simulink model "real_time_6"  (R2024b)
settings: Solver=FixedStepDiscrete  StartTime=0.0  StopTime=5  FixedStep=0.001  RelTol=1e-3
values from neighbouring files (symbols this model uses):
  AF = REG_disc.A    [code_ali.m]
  BF = REG_disc.B    [code_ali.m]
  CF = REG_disc.C    [code_ali.m]
  DF = REG_disc.D    [code_ali.m]
  K2 = K_robust(2:3)    [Pos_state_space.m]    (also in code_ali.m)
  KI = K_robust(1)    [Pos_state_space.m]    (also in code_ali.m)
  Nu = Ans(3,1)    [Pos_state_space.m]    (also in code_ali.m)
  Nx = Ans(1:2,1)    [Pos_state_space.m]    (also in code_ali.m)
  T_s = 0.001*10    (= 0.01)    [code_ali.m]
undefined symbols (not defined in the file or in its folder): degs2rpm, DiscIntNeverNeededParam, National_Instruments, PCI, rpm2rads
libraries: sldrtlib x3
settings Model: SimulationMode=external  ExtModeTrigDuration=1000001  Creator=galeazzolu  LastModifiedBy=galeazzolu
settings DataIOCC: ReturnWorkspaceOutputs=off
settings HardwareCC: ProdBitPerLong=64  ProdHWDeviceType=Intel->x86-64 (Linux 64)
settings RTWCC: Description=Simulink Desktop Real-Time  SystemTargetFile=sldrt.tlc  TemplateMakefile=sldrt.tmf  RTWCompilerOptimization=on
settings CodeAppCC: MaxIdLength=95
settings SimulinkDesktopRealTimeCC: TargetLibSuffix=_sldrt.a  TargetPreCompLibLocation=C:\Program Files\MATLAB\R2024b\toolbox\sldrt\lib\win64  ParMdlRefBuildCompliant=on

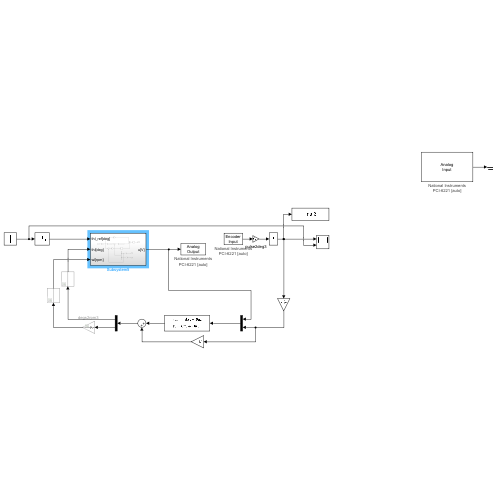
[thumbnail: Simulink's stored preview of the top-level diagram]
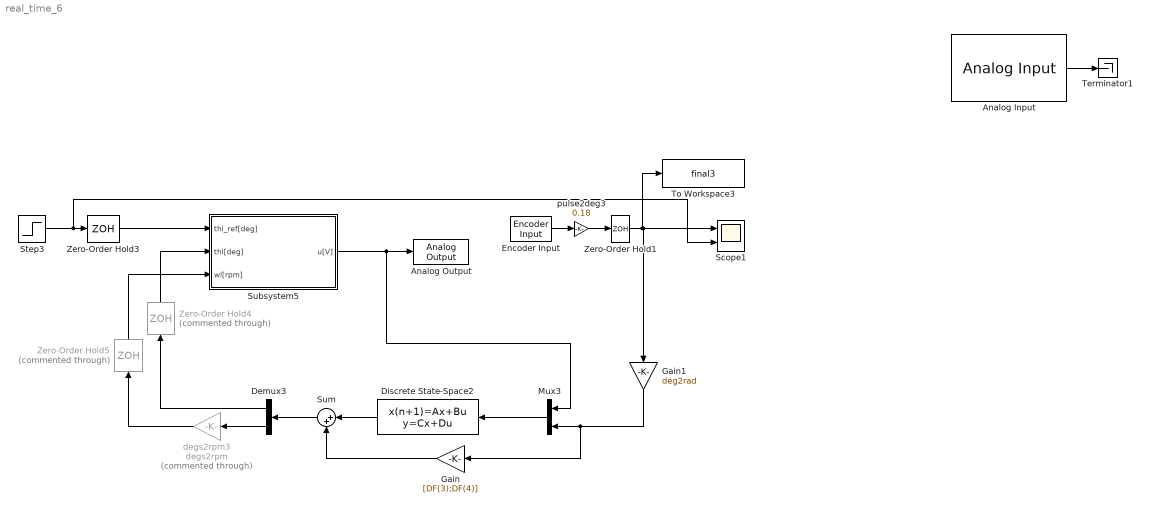
== system real_time_6 ==
  Analog Input : sldrtlib/Analog Input  SampleTime=-1  MaxMissedTicks=10  ShowMissedTicks=off  YieldWhenWaiting=off  DrvName=National_Instruments/PCI-6221  DrvAddress=4294967295  DrvOptions=[0 0 0 2 0]  Channels=[1,2]  RangeMode=1  VoltRange=1  DataType=1
      settings: AttributesFormatString=National Instruments\nPCI-6221 [auto]
  Analog Output : sldrtlib/Analog Output  SampleTime=-1  MaxMissedTicks=10  ShowMissedTicks=off  YieldWhenWaiting=off  DrvName=National_Instruments/PCI-6221  DrvAddress=4294967295  DrvOptions=[0 0 0 2 0]  Channels=1  RangeMode=1  VoltRange=1  InitialValue=0  FinalValue=0
      settings: AttributesFormatString=National Instruments\nPCI-6221 [auto]
  Demux3 : Demux  Outputs=2
  Discrete State-Space2 : DiscreteStateSpace  A=AF  B=BF  C=CF  D=[0,0;0,0]  SampleTime=T_s
  Encoder Input : sldrtlib/Encoder Input  SampleTime=-1  MaxMissedTicks=10  ShowMissedTicks=off  YieldWhenWaiting=off  DrvName=National_Instruments/PCI-6221  DrvAddress=4294967295  DrvOptions=[0 0 0 2 0]  Channels=1  QuadMode=3  IndexPulse=1  InputFilter=Inf  DataType=1
      settings: AttributesFormatString=National Instruments\nPCI-6221 [auto]
  Gain : Gain  Gain=[DF(3);DF(4)]
  Gain1 : Gain  Gain=deg2rad
  Mux3 : Mux  Inputs=2
  Scope1 : Scope  NumInputPorts=2
  Step3 : Step  Time=0  After=50  SampleTime=T_s
  Subsystem5 : Subsystem
  Sum : Sum  Inputs=|++
  Terminator1 : Terminator
  To Workspace3 : ToWorkspace  VariableName=final3  SaveFormat=Structure With Time  SampleTime=-1
  Zero-Order Hold1 : ZeroOrderHold  SampleTime=T_s
  Zero-Order Hold3 : ZeroOrderHold  SampleTime=T_s
  Zero-Order Hold4 : ZeroOrderHold  Commented=through  SampleTime=T_s
  Zero-Order Hold5 : ZeroOrderHold  Commented=through  SampleTime=T_s
  degs2rpm3 : Gain  Commented=through  Gain=degs2rpm
  pulse2deg3 : Gain  Gain=0.18
  wires:
  Analog Input/1 -> Terminator1/1
  Subsystem5/1(u[V]) -> Analog Output/1, Mux3/1
  Mux3/1 -> Discrete State-Space2/1
  pulse2deg3/1 -> Zero-Order Hold1/1
  Encoder Input/1 -> pulse2deg3/1
  Zero-Order Hold5/1 -> Subsystem5/3(wl[rpm])
  degs2rpm3/1 -> Zero-Order Hold5/1
  Zero-Order Hold3/1 -> Subsystem5/1(thl_ref[deg])
  Demux3/2 -> degs2rpm3/1
  Step3/1 -> Scope1/2, Zero-Order Hold3/1
  Zero-Order Hold4/1 -> Subsystem5/2(thl[deg])
  Discrete State-Space2/1 -> Sum/1
  Sum/1 -> Demux3/1
  Gain/1 -> Sum/2
  Gain1/1 -> Mux3/2, Gain/1
  Demux3/1 -> Zero-Order Hold4/1
  Zero-Order Hold1/1 -> Scope1/1, Gain1/1, To Workspace3/1

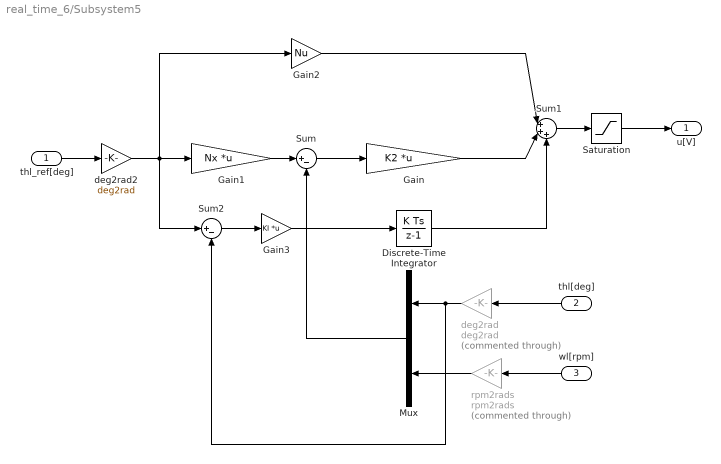
== system real_time_6/Subsystem5 ==
  thl_ref[deg] : Inport
  thl[deg] : Inport  Port=2
  wl[rpm] : Inport  Port=3
  Discrete-Time Integrator : DiscreteIntegrator  gainval=1  SampleTime=T_s  ICPrevOutput=DiscIntNeverNeededParam  ICPrevScaledInput=DiscIntNeverNeededParam
  Gain : Gain  Gain=K2  Multiplication=Matrix(K*u)
  Gain1 : Gain  Gain=Nx  Multiplication=Matrix(K*u)
  Gain2 : Gain  Gain=Nu
  Gain3 : Gain  Gain=KI  Multiplication=Matrix(K*u)
  Mux : Mux  Inputs=2
  Saturation : Saturate  UpperLimit=12  LowerLimit=-12
  Sum : Sum  Inputs=|+-
  Sum1 : Sum  Inputs=|+++
  Sum2 : Sum  Inputs=|+-
  deg2rad : Gain  Commented=through  Gain=deg2rad
  deg2rad2 : Gain  Gain=deg2rad
  rpm2rads : Gain  Commented=through  Gain=rpm2rads
  u[V] : Outport
  wires:
  thl[deg]/1 -> deg2rad/1
  wl[rpm]/1 -> rpm2rads/1
  deg2rad/1 -> Mux/1, Sum2/2
  rpm2rads/1 -> Mux/2
  Sum/1 -> Gain/1
  Gain1/1 -> Sum/1
  thl_ref[deg]/1 -> deg2rad2/1
  deg2rad2/1 -> Gain1/1, Sum2/1, Gain2/1
  Gain2/1 -> Sum1/1
  Gain/1 -> Sum1/2
  Sum1/1 -> Saturation/1
  Saturation/1 -> u[V]/1
  Sum2/1 -> Gain3/1
  Gain3/1 -> Discrete-Time Integrator/1
  Mux/1 -> Sum/2
  Discrete-Time Integrator/1 -> Sum1/3
